simulink model "THREE_MPPTSTEST"  (R2016b)
settings: Solver=VariableStepAuto  StartTime=0.0  StopTime=0.5  RelTol=1e-3
values from neighbouring files (symbols this model uses):
  A = 1.3    [PV_module_Code.m]
  Isc = 8.61    [PV_module_Code.m]
  Ki = 0.002    [PV_module_Code.m]
  Kv = -0.32    [PV_module_Code.m]
  Ns = 60    [PV_module_Code.m]
  Rp = 415    [PV_module_Code.m]
  Rs = 0.22    [PV_module_Code.m]
  Voc = 37.41    [PV_module_Code.m]
undefined symbols (not defined in the file or in its folder): sigbuilder_block
libraries: powerlib x45, powerlib_meascontrol x3, fuzblock x1
settings Model: Creator=adria  LastModifiedBy=adria

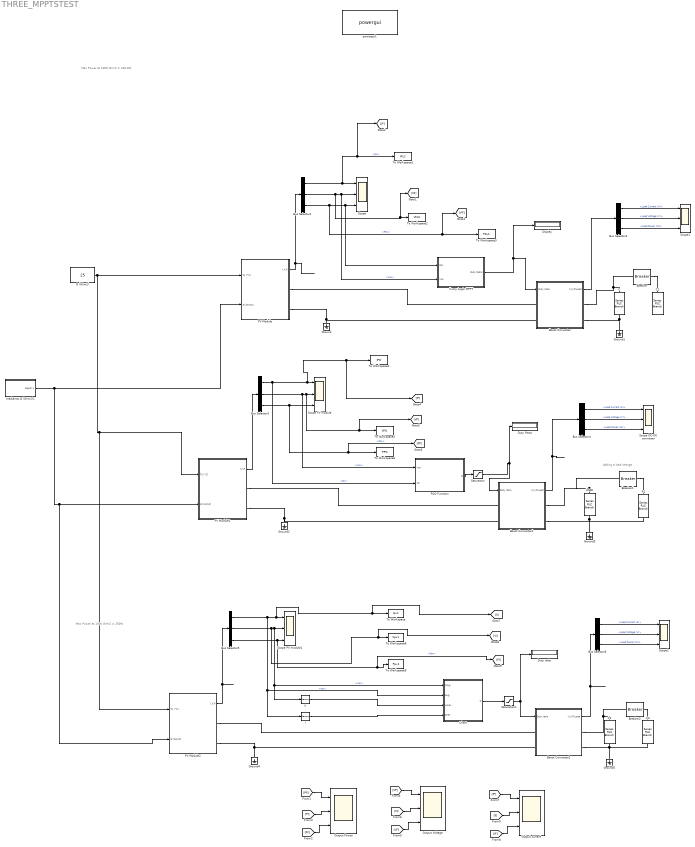
== system THREE_MPPTSTEST ==
  note: Max Power at 1000 W/m2 = 240.6W
  note: Adding a load change
  note: Max Power at 1000 W/m2 = 250W
  Boost Converter : Subsystem
  Boost Converter1 : Subsystem
  Boost Converter2 : Subsystem
  Breaker : powerlib/Elements/Breaker  InitialState=0  SwitchingTimes=[7]  External=off  BreakerResistance=0.00001  SnubberResistance=1e6  SnubberCapacitance=inf  Measurements=None  MoreParameters=on  NoBreakLoop=off
  Breaker1 : powerlib/Elements/Breaker  InitialState=0  SwitchingTimes=[5]  External=off  BreakerResistance=0.00001  SnubberResistance=1e6  SnubberCapacitance=inf  Measurements=None  MoreParameters=on  NoBreakLoop=off
  Breaker2 : powerlib/Elements/Breaker  InitialState=0  SwitchingTimes=[5]  External=off  BreakerResistance=0.00001  SnubberResistance=1e6  SnubberCapacitance=inf  Measurements=None  MoreParameters=on  NoBreakLoop=off
  Bus Selector1 : BusSelector  OutputSignals=Ipv,Vpv,Ppv
  Bus Selector2 : BusSelector  OutputSignals=Load Current (A),Load Voltage (V),Load Power (W)
  Bus Selector3 : BusSelector  OutputSignals=Ipv,Vpv,Ppv
  Bus Selector4 : BusSelector  OutputSignals=Load Current (A),Load Voltage (V),Load Power (W)
  Bus Selector5 : BusSelector  OutputSignals=Ipv,Vpv,Ppv
  Bus Selector6 : BusSelector  OutputSignals=Load Current (A),Load Voltage (V),Load Power (W)
  C : powerlib/Elements/Series RLC Branch  LConnTagsString=__new0  RConnTagsString=__new0  BranchType=R  Resistance=1000  Inductance=1e-3  SetiL0=off  InitialCurrent=0  Capacitance=19e-4  Setx0=off  InitialVoltage=0  Measurements=Branch voltage
  C1 : powerlib/Elements/Series RLC Branch  LConnTagsString=__new0  RConnTagsString=__new0  BranchType=R  Resistance=100  Inductance=1e-3  SetiL0=off  InitialCurrent=0  Capacitance=19e-4  Setx0=off  InitialVoltage=0  Measurements=Branch voltage
  C2 : powerlib/Elements/Series RLC Branch  LConnTagsString=__new0  RConnTagsString=__new0  BranchType=R  Resistance=100  Inductance=1e-3  SetiL0=off  InitialCurrent=0  Capacitance=19e-4  Setx0=off  InitialVoltage=0  Measurements=Branch voltage
  C3 : powerlib/Elements/Series RLC Branch  LConnTagsString=__new0  RConnTagsString=__new0  BranchType=R  Resistance=200  Inductance=1e-3  SetiL0=off  InitialCurrent=0  Capacitance=19e-4  Setx0=off  InitialVoltage=0  Measurements=Branch voltage
  Chart : Stateflow chart  TreatAsAtomicUnit=on
  Display : Display
  Duty Ratio : Display
  Duty ratio : Display
  Fuzzy Logic MPPT : Subsystem
  G (W/m2) : Constant  Value=25
  Ground{,1..5} (6 alike) : powerlib/Elements/Ground  LConnTagsString=a
  I : Memory
  Irradiance,G (W/m2)1 : Subsystem  Tag=STV Subsys  LoadFcn=sigbuilder_block('load');  StartFcn=sigbuilder_block('start');  StopFcn=sigbuilder_block('stop');  ClipboardFcn=sigbuilder_block('clipboard');  mask(Sigbuilder block){tuvar=[0:10]}
      mask help: Simulink:masks:SigbuilderBlock_MD
      mask init:
      | if ~strcmp(get_param(bdroot(gcbh),'SimulationStatus'),'stopped') tuvar = sigbuilder_block('maskInit'); end
      settings: CopyFcn=sigbuilder_block('copy');  DeleteFcn=sigbuilder_block('delete');  ModelCloseFcn=sigbuilder_block('modelClose');  PreSaveFcn=sigbuilder_block('preSave');  PauseFcn=sigbuilder_block('pause');  ContinueFcn=sigbuilder_block('continue');  NameChangeFcn=sigbuilder_block('namechange');  OpenFcn=sigbuilder_block('open',[484.8 30.6 470.4 453 ]);  CloseFcn=sigbuilder_block('close');
      mask Display: plot(0, 0, 100, 100,[2, 2, 32, 32, 2], [68, 8, 8, 68, 68],[32, 2], [38, 38], [32, 19, 2],[53, 60, 44], [32, 17, 17, 2],[16, 16, 31, 31]);txt = getActiveGroup(gcbh);text(2, 100, txt,'verticalAlignment', 'top');
  LOAD : powerlib/Elements/Series RLC Branch  LConnTagsString=__new0  RConnTagsString=__new0  BranchType=R  Resistance=100  Inductance=1e-3  SetiL0=off  InitialCurrent=0  Capacitance=19e-4  Setx0=off  InitialVoltage=0  Measurements=Branch voltage
  Output Power : Scope  NumInputPorts=3
  Output Voltage : Scope  NumInputPorts=3
  Output current : Scope  NumInputPorts=3
  P&O Function : MATLAB Function  TreatAsAtomicUnit=on
  PV Module : Subsystem
  PV Module1 : Subsystem
  PV Module2 : Subsystem
  R1 : powerlib/Elements/Series RLC Branch  LConnTagsString=__new0  RConnTagsString=__new0  BranchType=R  Resistance=200  Inductance=1e-3  SetiL0=off  InitialCurrent=0  Capacitance=19e-4  Setx0=off  InitialVoltage=0  Measurements=Branch voltage
  Saturation : Saturate  UpperLimit=1  LowerLimit=0.001  ZeroCross=off
  Saturation1 : Saturate  UpperLimit=1  LowerLimit=0.001  ZeroCross=off
  Scope : Scope  NumInputPorts=3
  Scope DC-DC converter : Scope  NumInputPorts=3
  Scope PV module1 : Scope  NumInputPorts=3
  Scope PV module : Scope  NumInputPorts=3
  Scope1 : Scope  NumInputPorts=3
  Scope2 : Scope  NumInputPorts=3
  To Workspace : ToWorkspace  VariableName=Ipv1  SampleTime=-1
  To Workspace1 : ToWorkspace  VariableName=IFLC  SampleTime=-1
  To Workspace2 : ToWorkspace  VariableName=VFLC  SampleTime=-1
  To Workspace3 : ToWorkspace  VariableName=PFLC  SampleTime=-1
  To Workspace4 : ToWorkspace  VariableName=IPO  SampleTime=-1
  To Workspace5 : ToWorkspace  VariableName=VPO  SampleTime=-1
  To Workspace6 : ToWorkspace  VariableName=PPO  SampleTime=-1
  To Workspace8 : ToWorkspace  VariableName=Vpv1  SampleTime=-1
  To Workspace9 : ToWorkspace  VariableName=Ppv1  SampleTime=-1
  V : Memory
  powergui1 : powerlib/powergui  Priority=1  SimulationMode=Discrete  SolverType=Tustin/Backward Euler (TBE)  SampleTime=0.000010  frequency=60  SPID=off  DisableSnubberDevices=off  DisableRonSwitches=off  DisableVfSwitches=off  SwTol=0  DisplayEquations=off  Interpol=off  ExternalGateDelay=off  methode=off  Ts=10  FunctionMessages=off  echomessages=off  HookPort=off  EnableUseOfTLC=off  x0status=blocks  frequencyindice=0  Pbase=100e6  ErrMax=1e-4  Iterations=50  UnitsV=kV  UnitsW=MW  buscounter=0  RestoreLinks=warning  ResistiveCurrentMeasurement=off  Frange=[0:2:500]  Ylog=off  Xlog=on  ShowGrid=off  save=off  variable=ZData  structure=0  ZoomFFT=off  StartTime=0.0  cycles=1  DisplayStyle=1  fundamental=60  FreqAxis=off  MaxFrequency=1000  frequencyindicesteady=1  RmsSteady=1  display=off
  wires:
  PV Module/1(I,V,P) -> Bus Selector1/1
  Bus Selector1/1 -> [IF], To Workspace1/1, Scope/1  "<Ipv>"
  Bus Selector1/2 -> [VF], To Workspace2/1, Fuzzy Logic MPPT/2(Vpv), Scope/2  "<Vpv>"
  Bus Selector1/3 -> [PF], To Workspace3/1, Fuzzy Logic MPPT/1(Ppv), Scope/3  "<Ppv>"
  Bus Selector2/1 -> Scope1/1  "<Load Current (A)>"
  Bus Selector2/2 -> Scope1/2  "<Load Voltage (V)>"
  Bus Selector2/3 -> Scope1/3  "<Load Power (W)>"
  Boost Converter/1((I,V,P)Load) -> Bus Selector2/1
  Fuzzy Logic MPPT/1(Duty Ratio) -> Display/1, Boost Converter/1("Duty ratio ")
  PV Module1/1(I,V,P) -> Bus Selector3/1
  Bus Selector3/1 -> P&O Function/2(Ipv), [IP], To Workspace4/1, Scope PV module/1  "<Ipv>"
  Bus Selector3/2 -> P&O Function/1(Vpv), [VP], To Workspace5/1, Scope PV module/2  "<Vpv>"
  Bus Selector3/3 -> [PP], To Workspace6/1, Scope PV module/3  "<Ppv>"
  Bus Selector4/1 -> Scope DC-DC converter/1  "<Load Current (A)>"
  Bus Selector4/2 -> Scope DC-DC converter/2  "<Load Voltage (V)>"
  Bus Selector4/3 -> Scope DC-DC converter/3  "<Load Power (W)>"
  Boost Converter1/1((I,V,P)Load) -> Bus Selector4/1
  P&O Function/1(D) -> Saturation/1
  Saturation/1 -> Duty Ratio/1, Boost Converter1/1("Duty ratio ")
  PV Module2/1(I,V,P) -> Bus Selector5/1
  Bus Selector5/1 -> I/1, Chart/2(Iavg), [II], To Workspace/1, Scope PV module1/1  "<Ipv>"
  Bus Selector6/1 -> Scope2/1  "<Load Current (A)>"
  Bus Selector6/2 -> Scope2/2  "<Load Voltage (V)>"
  Bus Selector6/3 -> Scope2/3  "<Load Power (W)>"
  Boost Converter2/1((I,V,P)Load) -> Bus Selector6/1
  Saturation1/1 -> Duty ratio/1, Boost Converter2/1("Duty ratio ")
  V/1 -> Chart/3(Vprev)
  I/1 -> Chart/4(Iprev)
  Chart/1(D) -> Saturation1/1
  Irradiance,G (W/m2)1/1(Signal 1) -> PV Module2/2(G (W/m2)), PV Module1/2(G (W/m2)), PV Module/2(G (W/m2))
  G (W/m2)/1 -> PV Module/1(Tc (°C)), PV Module2/1(Tc (°C)), PV Module1/1(Tc (°C))
  Bus Selector5/2 -> [VI], To Workspace8/1, V/1, Chart/1(Vavg), Scope PV module1/2  "<Vpv>"
  Bus Selector5/3 -> Scope PV module1/3, [PI], To Workspace9/1  "<Ppv>"
  [PF] -> Output Power/3
  [PI] -> Output Power/2
  [PP] -> Output Power/1
  [VF] -> Output Voltage/3
  [VI] -> Output Voltage/2
  [VP] -> Output Voltage/1
  [IF] -> Output current/3
  [II] -> Output current/2
  [IP] -> Output current/1
  connections:
  C/RConn1 -- Ground1/LConn1 -- Boost Converter/RConn2
  Boost Converter/LConn2 -- PV Module/RConn2 -- Ground/LConn1
  Breaker/LConn1 -- C/LConn1 -- Boost Converter/RConn1
  Breaker/RConn1 -- C1/LConn1
  PV Module/RConn1 -- Boost Converter/LConn1
  LOAD/RConn1 -- Boost Converter1/RConn2 -- Ground3/LConn1 -- R1/RConn1
  Ground2/LConn1 -- PV Module1/RConn2 -- Boost Converter1/LConn2
  LOAD/LConn1 -- Boost Converter1/RConn1 -- Breaker1/LConn1
  Breaker1/RConn1 -- R1/LConn1
  PV Module1/RConn1 -- Boost Converter1/LConn1
  Boost Converter2/RConn2 -- C2/RConn1 -- C3/RConn1 -- Ground5/LConn1
  PV Module2/RConn2 -- Boost Converter2/LConn2 -- Ground4/LConn1
  Breaker2/LConn1 -- C2/LConn1 -- Boost Converter2/RConn1
  Breaker2/RConn1 -- C3/LConn1
  PV Module2/RConn1 -- Boost Converter2/LConn1

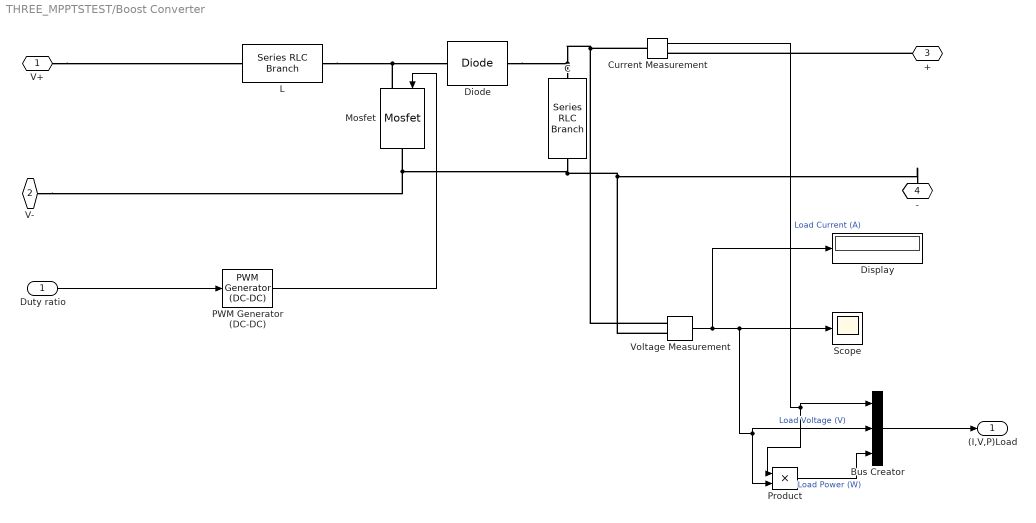
== system THREE_MPPTSTEST/Boost Converter ==
  "Duty ratio " : Inport
  Bus Creator : BusCreator  Inputs='Load Current (A)','Load Voltage (V)','Load Power (W)'
  C : powerlib/Elements/Series RLC Branch  LConnTagsString=__new0  RConnTagsString=__new0  BranchType=C  Resistance=1  Inductance=1e-3  SetiL0=off  InitialCurrent=0  Capacitance=50e-5  Setx0=off  InitialVoltage=0  Measurements=None
  Current Measurement : powerlib/Measurements/Current Measurement  PhasorSimulation=off  OutputType=Complex  PSBequivalent=0
  Diode : powerlib/Power Electronics/Diode  Ron=0.0001  Lon=0  Vf=0.8  IC=0  UseSnubber=off  Rs=500  Cs=250e-9  Measurements=off
  Display : Display
  L : powerlib/Elements/Series RLC Branch  LConnTagsString=__new0  RConnTagsString=__new0  BranchType=L  Resistance=1  Inductance=1e-3  SetiL0=off  InitialCurrent=0  Capacitance=1e-6  Setx0=off  InitialVoltage=0  Measurements=None
  Mosfet : powerlib/Power Electronics/Mosfet  Ron=0.0001  Lon=0  Rd=0.0001  Vfd=0  IC=0  Rs=1e5  Cs=inf  Measurements=off
  PWM Generator (DC-DC) : powerlib_meascontrol/Pulse & Signal Generators/PWM Generator (DC-DC)  Fsw=1000  Ts=0
  Product : Product
  Scope : Scope
  Voltage Measurement : powerlib/Measurements/Voltage Measurement  PhasorSimulation=off  OutputType=Complex  PSBequivalent=0
  V+ : PMIOPort  Port=1  Side=Left
  V- : PMIOPort  Port=2  Side=Left
  + : PMIOPort  Port=3  Side=Right
  - : PMIOPort  Port=4  Side=Right
  (I,V,P)Load : Outport
  wires:
  PWM Generator (DC-DC)/1 -> Mosfet/1
  Voltage Measurement/1 -> Display/1, Product/2, Bus Creator/2, Scope/1  "Load Voltage (V)"
  "Duty ratio "/1 -> PWM Generator (DC-DC)/1
  Current Measurement/1 -> Product/1, Bus Creator/1  "Load Current (A)"
  Product/1 -> Bus Creator/3  "Load Power (W)"
  Bus Creator/1 -> (I,V,P)Load/1
  connections:
  V+/RConn1 -- L/LConn1
  L/RConn1 -- Mosfet/LConn1 -- Diode/LConn1
  +/RConn1 -- Current Measurement/RConn1
  -/RConn1 -- Voltage Measurement/LConn2 -- V-/RConn1 -- Mosfet/RConn1 -- C/RConn1
  Diode/RConn1 -- Current Measurement/LConn1 -- Voltage Measurement/LConn1 -- C/LConn1

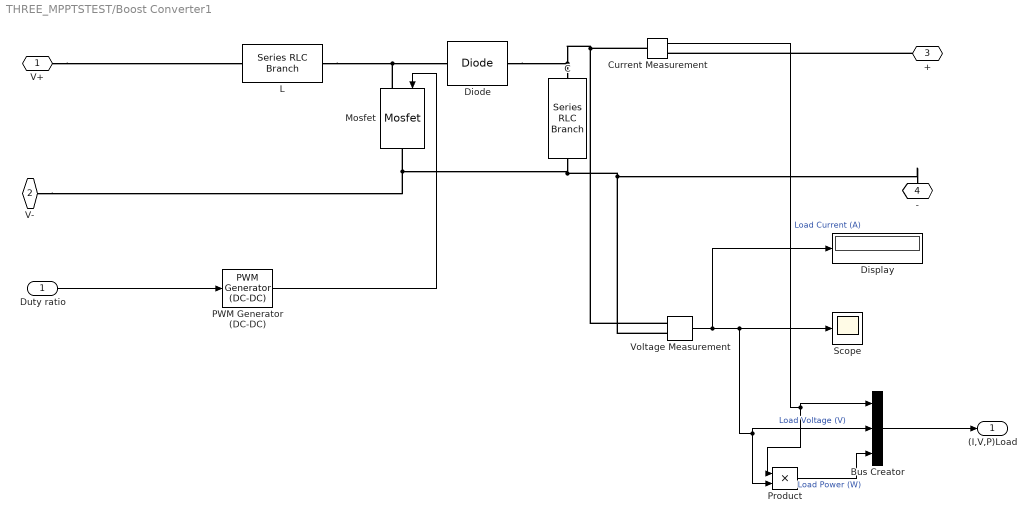
== system THREE_MPPTSTEST/Boost Converter1 ==
  "Duty ratio " : Inport
  Bus Creator : BusCreator  Inputs='Load Current (A)','Load Voltage (V)','Load Power (W)'
  C : powerlib/Elements/Series RLC Branch  LConnTagsString=__new0  RConnTagsString=__new0  BranchType=C  Resistance=1  Inductance=1e-3  SetiL0=off  InitialCurrent=0  Capacitance=50e-5  Setx0=off  InitialVoltage=0  Measurements=None
  Current Measurement : powerlib/Measurements/Current Measurement  PhasorSimulation=off  OutputType=Complex  PSBequivalent=0
  Diode : powerlib/Power Electronics/Diode  Ron=0.0001  Lon=0  Vf=0.8  IC=0  UseSnubber=off  Rs=500  Cs=250e-9  Measurements=off
  Display : Display
  L : powerlib/Elements/Series RLC Branch  LConnTagsString=__new0  RConnTagsString=__new0  BranchType=L  Resistance=1  Inductance=1e-3  SetiL0=off  InitialCurrent=0  Capacitance=1e-6  Setx0=off  InitialVoltage=0  Measurements=None
  Mosfet : powerlib/Power Electronics/Mosfet  Ron=0.0001  Lon=0  Rd=0.0001  Vfd=0  IC=0  Rs=1e5  Cs=inf  Measurements=off
  PWM Generator (DC-DC) : powerlib_meascontrol/Pulse & Signal Generators/PWM Generator (DC-DC)  Fsw=1000  Ts=0
  Product : Product
  Scope : Scope
  Voltage Measurement : powerlib/Measurements/Voltage Measurement  PhasorSimulation=off  OutputType=Complex  PSBequivalent=0
  V+ : PMIOPort  Port=1  Side=Left
  V- : PMIOPort  Port=2  Side=Left
  + : PMIOPort  Port=3  Side=Right
  - : PMIOPort  Port=4  Side=Right
  (I,V,P)Load : Outport
  wires:
  PWM Generator (DC-DC)/1 -> Mosfet/1
  Voltage Measurement/1 -> Display/1, Product/2, Bus Creator/2, Scope/1  "Load Voltage (V)"
  "Duty ratio "/1 -> PWM Generator (DC-DC)/1
  Current Measurement/1 -> Product/1, Bus Creator/1  "Load Current (A)"
  Product/1 -> Bus Creator/3  "Load Power (W)"
  Bus Creator/1 -> (I,V,P)Load/1
  connections:
  V+/RConn1 -- L/LConn1
  L/RConn1 -- Mosfet/LConn1 -- Diode/LConn1
  +/RConn1 -- Current Measurement/RConn1
  -/RConn1 -- Voltage Measurement/LConn2 -- V-/RConn1 -- Mosfet/RConn1 -- C/RConn1
  Diode/RConn1 -- Current Measurement/LConn1 -- Voltage Measurement/LConn1 -- C/LConn1

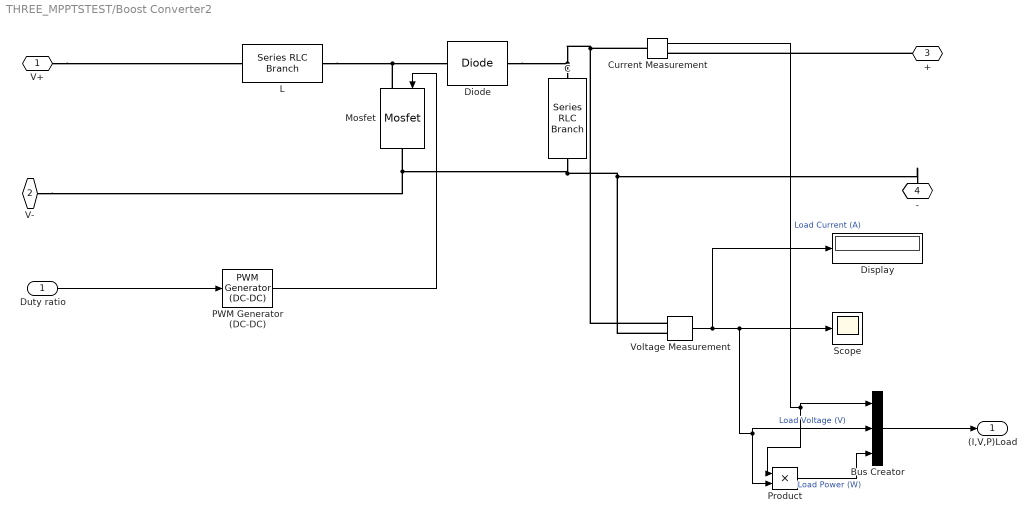
== system THREE_MPPTSTEST/Boost Converter2 ==
  "Duty ratio " : Inport
  Bus Creator : BusCreator  Inputs='Load Current (A)','Load Voltage (V)','Load Power (W)'
  C : powerlib/Elements/Series RLC Branch  LConnTagsString=__new0  RConnTagsString=__new0  BranchType=C  Resistance=1  Inductance=1e-3  SetiL0=off  InitialCurrent=0  Capacitance=50e-5  Setx0=off  InitialVoltage=0  Measurements=None
  Current Measurement : powerlib/Measurements/Current Measurement  PhasorSimulation=off  OutputType=Complex  PSBequivalent=0
  Diode : powerlib/Power Electronics/Diode  Ron=0.001  Lon=0  Vf=0.8  IC=0  UseSnubber=off  Rs=500  Cs=250e-9  Measurements=off
  Display : Display
  L : powerlib/Elements/Series RLC Branch  LConnTagsString=__new0  RConnTagsString=__new0  BranchType=L  Resistance=1  Inductance=1e-3  SetiL0=off  InitialCurrent=0  Capacitance=1e-6  Setx0=off  InitialVoltage=0  Measurements=None
  Mosfet : powerlib/Power Electronics/Mosfet  Ron=0.0001  Lon=0  Rd=0.0001  Vfd=0  IC=0  Rs=1e5  Cs=inf  Measurements=off
  PWM Generator (DC-DC) : powerlib_meascontrol/Pulse & Signal Generators/PWM Generator (DC-DC)  Fsw=1000  Ts=0
  Product : Product
  Scope : Scope
  Voltage Measurement : powerlib/Measurements/Voltage Measurement  PhasorSimulation=off  OutputType=Complex  PSBequivalent=0
  V+ : PMIOPort  Port=1  Side=Left
  V- : PMIOPort  Port=2  Side=Left
  + : PMIOPort  Port=3  Side=Right
  - : PMIOPort  Port=4  Side=Right
  (I,V,P)Load : Outport
  wires:
  PWM Generator (DC-DC)/1 -> Mosfet/1
  Voltage Measurement/1 -> Display/1, Product/2, Bus Creator/2, Scope/1  "Load Voltage (V)"
  "Duty ratio "/1 -> PWM Generator (DC-DC)/1
  Current Measurement/1 -> Product/1, Bus Creator/1  "Load Current (A)"
  Product/1 -> Bus Creator/3  "Load Power (W)"
  Bus Creator/1 -> (I,V,P)Load/1
  connections:
  V+/RConn1 -- L/LConn1
  L/RConn1 -- Mosfet/LConn1 -- Diode/LConn1
  +/RConn1 -- Current Measurement/RConn1
  -/RConn1 -- Voltage Measurement/LConn2 -- V-/RConn1 -- Mosfet/RConn1 -- C/RConn1
  Diode/RConn1 -- Current Measurement/LConn1 -- Voltage Measurement/LConn1 -- C/LConn1

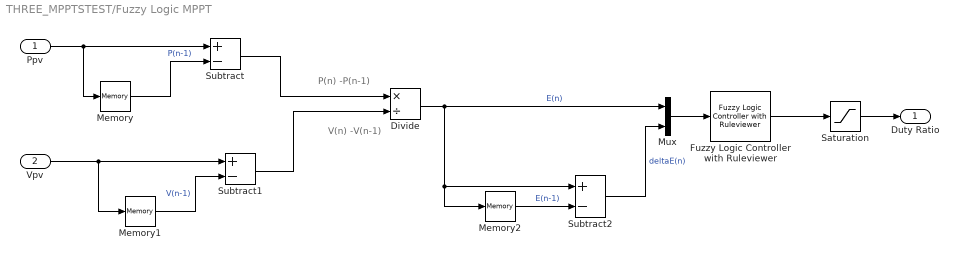
== system THREE_MPPTSTEST/Fuzzy Logic MPPT ==
  note: P(n) -P(n-1)
  note: V(n) -V(n-1)
  Ppv : Inport
  Vpv : Inport  Port=2
  Divide : Product  Inputs=*/
  Fuzzy Logic Controller with Ruleviewer : fuzblock/Fuzzy Logic  Controller  with Ruleviewer  fismatrix=MPPT8  Ts=1
  Memory : Memory  InheritSampleTime=on
  Memory1 : Memory  InheritSampleTime=on
  Memory2 : Memory
  Mux : Mux  Inputs=2
  Saturation : Saturate  UpperLimit=1  LowerLimit=0  LinearizeAsGain=off  ZeroCross=off
  Subtract : Sum  Inputs=+-
  Subtract1 : Sum  Inputs=+-
  Subtract2 : Sum  Inputs=+-
  Duty Ratio : Outport
  wires:
  Ppv/1 -> Subtract/1, Memory/1
  Mux/1 -> Fuzzy Logic Controller with Ruleviewer/1
  Divide/1 -> Subtract2/1, Memory2/1, Mux/1  "E(n)"
  Memory2/1 -> Subtract2/2  "E(n-1)"
  Subtract2/1 -> Mux/2  "deltaE(n)"
  Memory/1 -> Subtract/2  "P(n-1)"
  Vpv/1 -> Memory1/1, Subtract1/1
  Memory1/1 -> Subtract1/2  "V(n-1)"
  Saturation/1 -> Duty Ratio/1
  Subtract1/1 -> Divide/2
  Subtract/1 -> Divide/1
  Fuzzy Logic Controller with Ruleviewer/1 -> Saturation/1

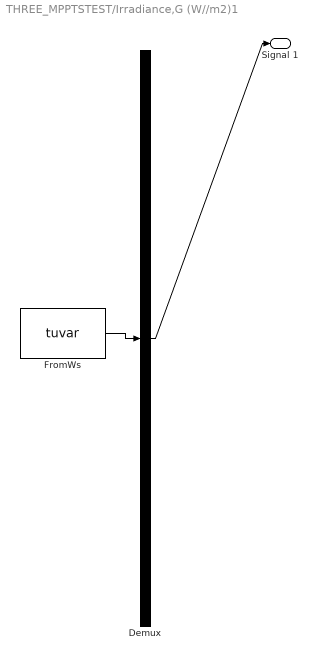
== system THREE_MPPTSTEST/Irradiance,G (W//m2)1 ==
  Demux : Demux  Tag=STV Demux  Outputs=1
  FromWs : FromWorkspace  Tag=STV FromWs  VariableName=tuvar  SampleTime=0
      SigBuilderData=|
      | common.afterFinalStr = 'Extrapolate'
      | common.sampleTime = 0
      | dataSet.timeRange = [0 10]
      | dataSet.name = 'Irradiance Variation Pattern'
      | sbobj.Groups.Name = 'Irradiance Variation Pattern'
      | sbobj.Groups.Signals.Name = 'Signal 1'
      | sbobj.Groups.Signals.XData = [0 0.2 0.2 0.3 0.3 0.8 0.8 0.9 2.4 2.4 3.6 3.6 10]
      | sbobj.Groups.Signals.YData = [1000 1000 300 300 1000 1000 995 995 995 575 1 0 0]
  Signal 1 : Outport  Tag=STV Outport
  wires:
  FromWs/1 -> Demux/1
  Demux/1 -> Signal 1/1

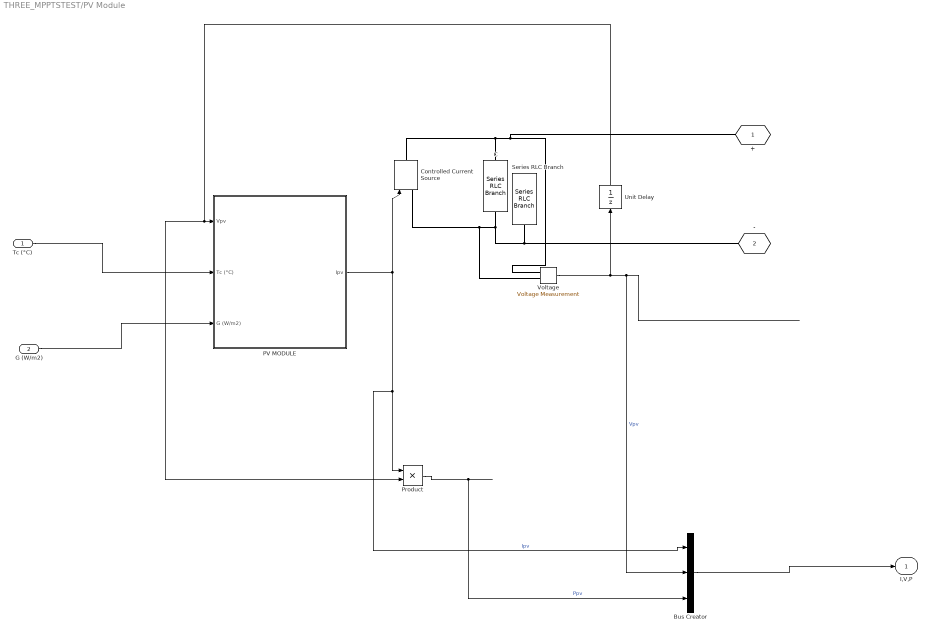
== system THREE_MPPTSTEST/PV Module ==
  Tc (°C) : Inport
  G (W/m2) : Inport  Port=2
  Bus Creator : BusCreator  Inputs='Ipv','Vpv','Ppv'
  C : powerlib/Elements/Series RLC Branch  LConnTagsString=__new0  RConnTagsString=__new0  BranchType=C  Resistance=10  Inductance=1e-3  SetiL0=off  InitialCurrent=0  Capacitance=30e-4  Setx0=off  InitialVoltage=0  Measurements=Branch voltage
  Controlled Current Source : powerlib/Electrical Sources/Controlled Current Source  Initialize=on  Source_Type=DC  Amplitude=0  Phase=0  Frequency=0  Measurements=None
  PV MODULE : Subsystem
  Product : Product
  Series RLC Branch : powerlib/Elements/Series RLC Branch  LConnTagsString=__new0  RConnTagsString=__new0  BranchType=R  Resistance=1000  Inductance=1e-3  SetiL0=off  InitialCurrent=0  Capacitance=1e-6  Setx0=off  InitialVoltage=0  Measurements=None
  Unit Delay : UnitDelay  SampleTime=-1
  "Voltage " : powerlib/Measurements/Voltage Measurement  PhasorSimulation=off  OutputType=Complex  PSBequivalent=0
  + : PMIOPort  Port=1  Side=Right
  - : PMIOPort  Port=2  Side=Right
  I,V,P : Outport
  wires:
  Product/1 -> Bus Creator/3  "Ppv"
  Tc (°C)/1 -> PV MODULE/2("Tc (°C) ")
  G (W/m2)/1 -> PV MODULE/3(G (W/m2))
  "Voltage "/1 -> Unit Delay/1, Bus Creator/2  "Vpv"
  PV MODULE/1(Ipv) -> Controlled Current Source/1, Bus Creator/1, Product/1  "Ipv"
  Bus Creator/1 -> I,V,P/1
  Unit Delay/1 -> Product/2, PV MODULE/1(Vpv)
  connections:
  Controlled Current Source/LConn1 -- Series RLC Branch/RConn1 -- -/RConn1 -- C/RConn1 -- "Voltage "/LConn2
  Controlled Current Source/RConn1 -- C/LConn1 -- "Voltage "/LConn1 -- +/RConn1

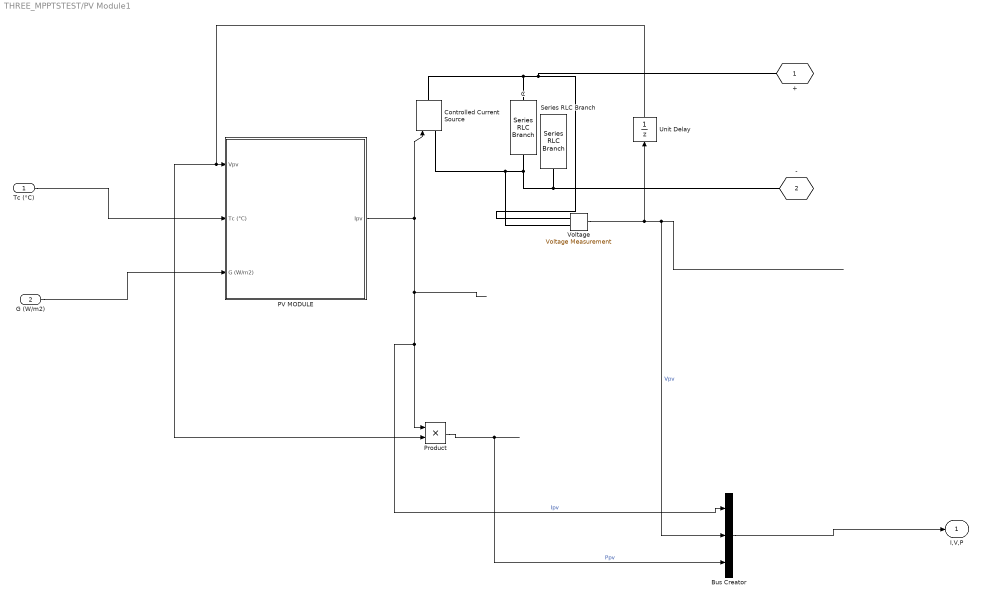
== system THREE_MPPTSTEST/PV Module1 ==
  Tc (°C) : Inport
  G (W/m2) : Inport  Port=2
  Bus Creator : BusCreator  Inputs='Ipv','Vpv','Ppv'
  C : powerlib/Elements/Series RLC Branch  LConnTagsString=__new0  RConnTagsString=__new0  BranchType=C  Resistance=10  Inductance=1e-3  SetiL0=off  InitialCurrent=0  Capacitance=30e-4  Setx0=off  InitialVoltage=0  Measurements=Branch voltage
  Controlled Current Source : powerlib/Electrical Sources/Controlled Current Source  Initialize=on  Source_Type=AC  Amplitude=0  Phase=0  Frequency=0  Measurements=None
  PV MODULE : Subsystem
  Product : Product
  Series RLC Branch : powerlib/Elements/Series RLC Branch  LConnTagsString=__new0  RConnTagsString=__new0  BranchType=R  Resistance=1000  Inductance=1e-3  SetiL0=off  InitialCurrent=0  Capacitance=1e-6  Setx0=off  InitialVoltage=0  Measurements=None
  Unit Delay : UnitDelay  SampleTime=-1
  "Voltage " : powerlib/Measurements/Voltage Measurement  PhasorSimulation=off  OutputType=Complex  PSBequivalent=0
  + : PMIOPort  Port=1  Side=Right
  - : PMIOPort  Port=2  Side=Right
  I,V,P : Outport
  wires:
  Product/1 -> Bus Creator/3  "Ppv"
  Tc (°C)/1 -> PV MODULE/2("Tc (°C) ")
  G (W/m2)/1 -> PV MODULE/3(G (W/m2))
  "Voltage "/1 -> Unit Delay/1, Bus Creator/2  "Vpv"
  PV MODULE/1(Ipv) -> Controlled Current Source/1, Bus Creator/1, Product/1  "Ipv"
  Bus Creator/1 -> I,V,P/1
  Unit Delay/1 -> Product/2, PV MODULE/1(Vpv)
  connections:
  Controlled Current Source/LConn1 -- Series RLC Branch/RConn1 -- -/RConn1 -- C/RConn1 -- "Voltage "/LConn2
  Controlled Current Source/RConn1 -- C/LConn1 -- "Voltage "/LConn1 -- +/RConn1

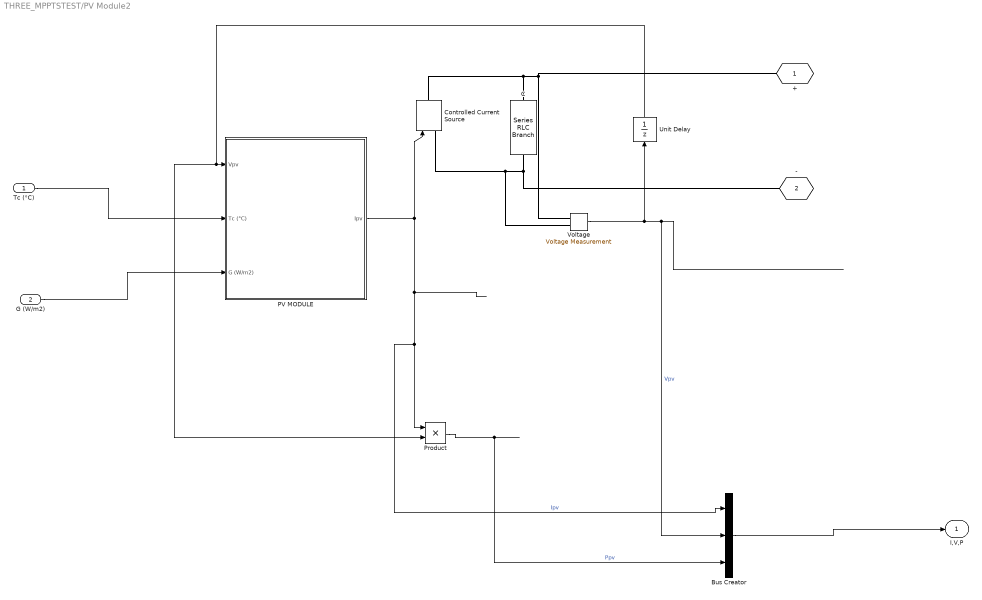
== system THREE_MPPTSTEST/PV Module2 ==
  Tc (°C) : Inport
  G (W/m2) : Inport  Port=2
  Bus Creator : BusCreator  Inputs='Ipv','Vpv','Ppv'
  C : powerlib/Elements/Series RLC Branch  LConnTagsString=__new0  RConnTagsString=__new0  BranchType=C  Resistance=10  Inductance=1e-3  SetiL0=off  InitialCurrent=0  Capacitance=30e-4  Setx0=off  InitialVoltage=0  Measurements=Branch voltage
  Controlled Current Source : powerlib/Electrical Sources/Controlled Current Source  Initialize=on  Source_Type=AC  Amplitude=0  Phase=0  Frequency=0  Measurements=None
  PV MODULE : Subsystem
  Product : Product
  Unit Delay : UnitDelay  SampleTime=-1
  "Voltage " : powerlib/Measurements/Voltage Measurement  PhasorSimulation=off  OutputType=Complex  PSBequivalent=0
  + : PMIOPort  Port=1  Side=Right
  - : PMIOPort  Port=2  Side=Right
  I,V,P : Outport
  wires:
  Product/1 -> Bus Creator/3  "Ppv"
  Tc (°C)/1 -> PV MODULE/2("Tc (°C) ")
  G (W/m2)/1 -> PV MODULE/3(G (W/m2))
  "Voltage "/1 -> Unit Delay/1, Bus Creator/2  "Vpv"
  PV MODULE/1(Ipv) -> Controlled Current Source/1, Bus Creator/1, Product/1  "Ipv"
  Bus Creator/1 -> I,V,P/1
  Unit Delay/1 -> Product/2, PV MODULE/1(Vpv)
  connections:
  Controlled Current Source/LConn1 -- -/RConn1 -- C/RConn1 -- "Voltage "/LConn2
  Controlled Current Source/RConn1 -- C/LConn1 -- +/RConn1 -- "Voltage "/LConn1

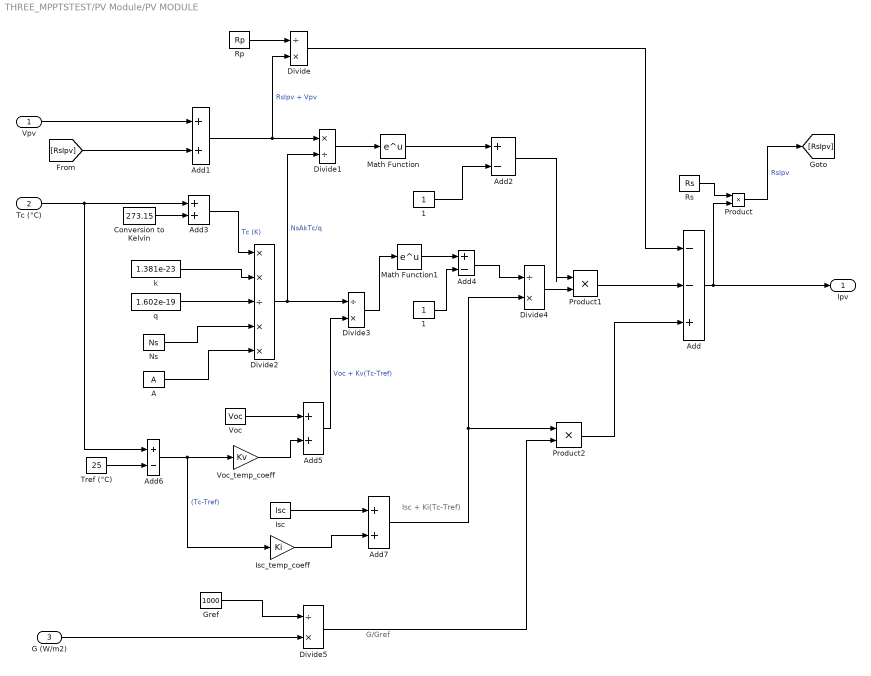
== system THREE_MPPTSTEST/PV Module/PV MODULE ==
  note: G/Gref
  note: Isc + Ki(Tc-Tref)
  Vpv : Inport
  "Tc (°C) " : Inport  Port=2
  G (W/m2) : Inport  Port=3
  " 1" : Constant
  " Gref " : Constant  Value=1000
  " Tref (°C)" : Constant  Value=25
  " Voc" : Constant  Value=Voc
  1 : Constant
  A : Constant  Value=A
  Add : Sum  Inputs=--+
  Add{1,3,5,7} (4 alike) : Sum
  Add2 : Sum  Inputs=+-
  Add4 : Sum  Inputs=+-
  Add6 : Sum  Inputs=+-
  Conversion to Kelvin : Constant  Value=273.15
  Divide{,3..5} (4 alike) : Product  Inputs=/*
  Divide1 : Product  Inputs=*/
  Divide2 : Product  Inputs=**/**
  Isc : Constant  Value=Isc
  "Isc_temp_coeff " : Gain  Gain=Ki
  Math Function : Math  SaturateOnIntegerOverflow=on
  Math Function1 : Math  SaturateOnIntegerOverflow=on
  Ns : Constant  Value=Ns
  Product : Product
  Product1 : Product
  Product2 : Product
  Rp : Constant  Value=Rp
  Rs : Constant  Value=Rs
  Voc_temp_coeff : Gain  Gain=Kv
  k : Constant  Value=1.381e-23
  "q " : Constant  Value=1.602e-19
  Ipv : Outport
  wires:
  A/1 -> Divide2/5
  Vpv/1 -> Add1/1
  Rp/1 -> Divide/1
  Add/1 -> Ipv/1, Product/2
  Product/1 -> [RsIpv]  "RsIpv"
  Divide/1 -> Add/1
  Add1/1 -> Divide1/1, Divide/2  "RsIpv + Vpv"
  Rs/1 -> Product/1
  Product2/1 -> Add/3
  Divide2/1 -> Divide3/1, Divide1/2  "NsAkTc/q"
  k/1 -> Divide2/2
  Math Function1/1 -> Add4/1
  " Voc"/1 -> Add5/1
  Divide4/1 -> Product1/2
  Add2/1 -> Product1/1
  Math Function/1 -> Add2/1
  Divide3/1 -> Math Function1/1
  "q "/1 -> Divide2/3
  Add6/1 -> "Isc_temp_coeff "/1, Voc_temp_coeff/1  "(Tc-Tref)"
  " 1"/1 -> Add4/2
  Isc/1 -> Add7/1
  Add7/1 -> Product2/1, Divide4/2
  "Tc (°C) "/1 -> Add6/1, Add3/1
  Add4/1 -> Divide4/1
  Product1/1 -> Add/2
  Divide5/1 -> Product2/2
  Conversion to Kelvin/1 -> Add3/2
  Add5/1 -> Divide3/2  "Voc + Kv(Tc-Tref)"
  "Isc_temp_coeff "/1 -> Add7/2
  Divide1/1 -> Math Function/1
  " Gref "/1 -> Divide5/1
  " Tref (°C)"/1 -> Add6/2
  G (W/m2)/1 -> Divide5/2
  Voc_temp_coeff/1 -> Add5/2
  Add3/1 -> Divide2/1  "Tc (K)"
  Ns/1 -> Divide2/4
  1/1 -> Add2/2
  [RsIpv] -> Add1/2

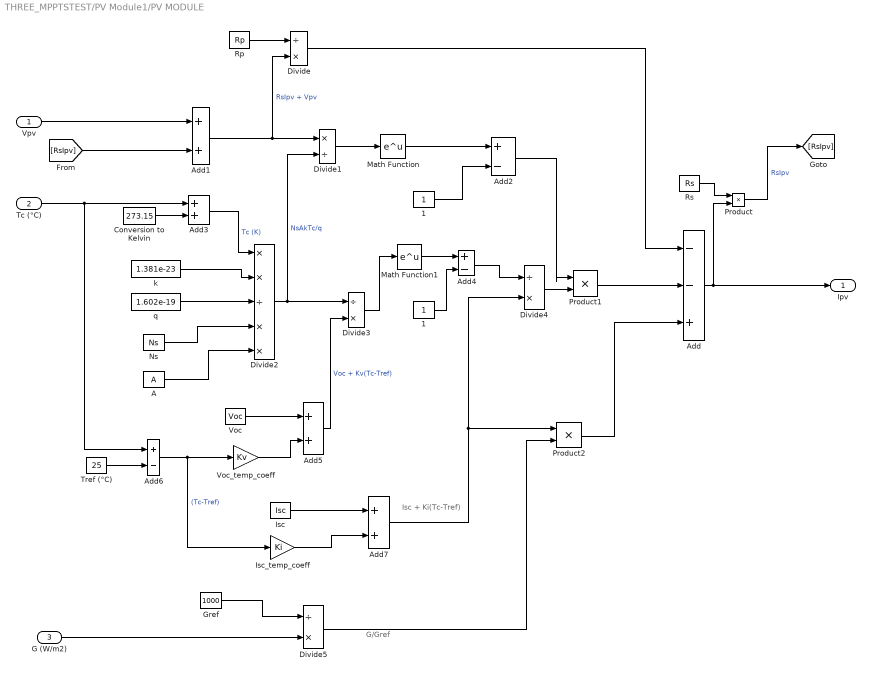
== system THREE_MPPTSTEST/PV Module1/PV MODULE ==
  note: G/Gref
  note: Isc + Ki(Tc-Tref)
  Vpv : Inport
  "Tc (°C) " : Inport  Port=2
  G (W/m2) : Inport  Port=3
  " 1" : Constant
  " Gref " : Constant  Value=1000
  " Tref (°C)" : Constant  Value=25
  " Voc" : Constant  Value=Voc
  1 : Constant
  A : Constant  Value=A
  Add : Sum  Inputs=--+
  Add{1,3,5,7} (4 alike) : Sum
  Add2 : Sum  Inputs=+-
  Add4 : Sum  Inputs=+-
  Add6 : Sum  Inputs=+-
  Conversion to Kelvin : Constant  Value=273.15
  Divide{,3..5} (4 alike) : Product  Inputs=/*
  Divide1 : Product  Inputs=*/
  Divide2 : Product  Inputs=**/**
  Isc : Constant  Value=Isc
  "Isc_temp_coeff " : Gain  Gain=Ki
  Math Function : Math  SaturateOnIntegerOverflow=on
  Math Function1 : Math  SaturateOnIntegerOverflow=on
  Ns : Constant  Value=Ns
  Product : Product
  Product1 : Product
  Product2 : Product
  Rp : Constant  Value=Rp
  Rs : Constant  Value=Rs
  Voc_temp_coeff : Gain  Gain=Kv
  k : Constant  Value=1.381e-23
  "q " : Constant  Value=1.602e-19
  Ipv : Outport
  wires:
  A/1 -> Divide2/5
  Vpv/1 -> Add1/1
  Rp/1 -> Divide/1
  Add/1 -> Ipv/1, Product/2
  Product/1 -> [RsIpv]  "RsIpv"
  Divide/1 -> Add/1
  Add1/1 -> Divide1/1, Divide/2  "RsIpv + Vpv"
  Rs/1 -> Product/1
  Product2/1 -> Add/3
  Divide2/1 -> Divide3/1, Divide1/2  "NsAkTc/q"
  k/1 -> Divide2/2
  Math Function1/1 -> Add4/1
  " Voc"/1 -> Add5/1
  Divide4/1 -> Product1/2
  Add2/1 -> Product1/1
  Math Function/1 -> Add2/1
  Divide3/1 -> Math Function1/1
  "q "/1 -> Divide2/3
  Add6/1 -> "Isc_temp_coeff "/1, Voc_temp_coeff/1  "(Tc-Tref)"
  " 1"/1 -> Add4/2
  Isc/1 -> Add7/1
  Add7/1 -> Product2/1, Divide4/2
  "Tc (°C) "/1 -> Add6/1, Add3/1
  Add4/1 -> Divide4/1
  Product1/1 -> Add/2
  Divide5/1 -> Product2/2
  Conversion to Kelvin/1 -> Add3/2
  Add5/1 -> Divide3/2  "Voc + Kv(Tc-Tref)"
  "Isc_temp_coeff "/1 -> Add7/2
  Divide1/1 -> Math Function/1
  " Gref "/1 -> Divide5/1
  " Tref (°C)"/1 -> Add6/2
  G (W/m2)/1 -> Divide5/2
  Voc_temp_coeff/1 -> Add5/2
  Add3/1 -> Divide2/1  "Tc (K)"
  Ns/1 -> Divide2/4
  1/1 -> Add2/2
  [RsIpv] -> Add1/2

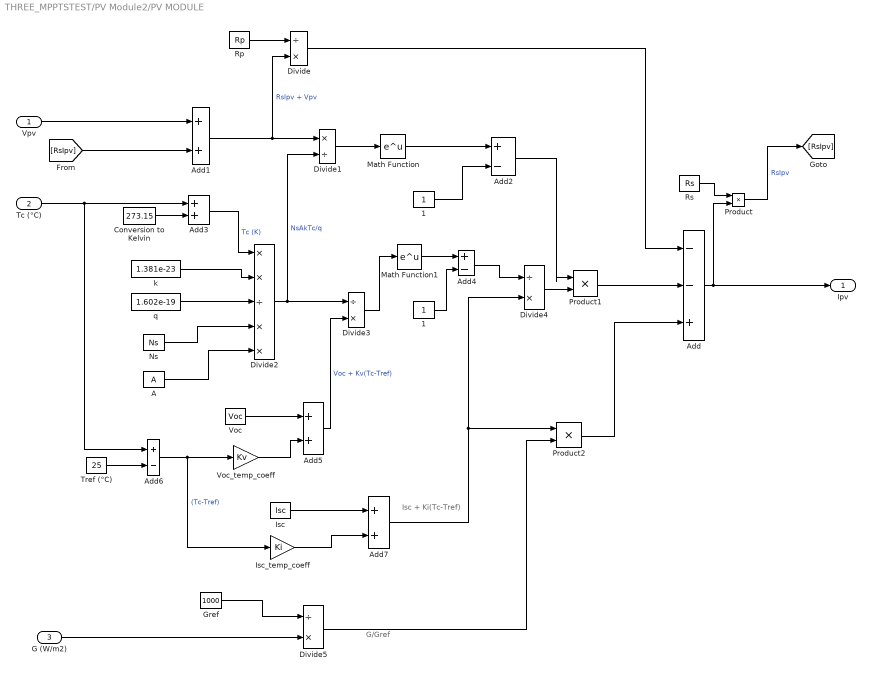
== system THREE_MPPTSTEST/PV Module2/PV MODULE ==
  note: G/Gref
  note: Isc + Ki(Tc-Tref)
  Vpv : Inport
  "Tc (°C) " : Inport  Port=2
  G (W/m2) : Inport  Port=3
  " 1" : Constant
  " Gref " : Constant  Value=1000
  " Tref (°C)" : Constant  Value=25
  " Voc" : Constant  Value=Voc
  1 : Constant
  A : Constant  Value=A
  Add : Sum  Inputs=--+
  Add{1,3,5,7} (4 alike) : Sum
  Add2 : Sum  Inputs=+-
  Add4 : Sum  Inputs=+-
  Add6 : Sum  Inputs=+-
  Conversion to Kelvin : Constant  Value=273.15
  Divide{,3..5} (4 alike) : Product  Inputs=/*
  Divide1 : Product  Inputs=*/
  Divide2 : Product  Inputs=**/**
  Isc : Constant  Value=Isc
  "Isc_temp_coeff " : Gain  Gain=Ki
  Math Function : Math  SaturateOnIntegerOverflow=on
  Math Function1 : Math  SaturateOnIntegerOverflow=on
  Ns : Constant  Value=Ns
  Product : Product
  Product1 : Product
  Product2 : Product
  Rp : Constant  Value=Rp
  Rs : Constant  Value=Rs
  Voc_temp_coeff : Gain  Gain=Kv
  k : Constant  Value=1.381e-23
  "q " : Constant  Value=1.602e-19
  Ipv : Outport
  wires:
  A/1 -> Divide2/5
  Vpv/1 -> Add1/1
  Rp/1 -> Divide/1
  Add/1 -> Ipv/1, Product/2
  Product/1 -> [RsIpv]  "RsIpv"
  Divide/1 -> Add/1
  Add1/1 -> Divide1/1, Divide/2  "RsIpv + Vpv"
  Rs/1 -> Product/1
  Product2/1 -> Add/3
  Divide2/1 -> Divide3/1, Divide1/2  "NsAkTc/q"
  k/1 -> Divide2/2
  Math Function1/1 -> Add4/1
  " Voc"/1 -> Add5/1
  Divide4/1 -> Product1/2
  Add2/1 -> Product1/1
  Math Function/1 -> Add2/1
  Divide3/1 -> Math Function1/1
  "q "/1 -> Divide2/3
  Add6/1 -> "Isc_temp_coeff "/1, Voc_temp_coeff/1  "(Tc-Tref)"
  " 1"/1 -> Add4/2
  Isc/1 -> Add7/1
  Add7/1 -> Product2/1, Divide4/2
  "Tc (°C) "/1 -> Add6/1, Add3/1
  Add4/1 -> Divide4/1
  Product1/1 -> Add/2
  Divide5/1 -> Product2/2
  Conversion to Kelvin/1 -> Add3/2
  Add5/1 -> Divide3/2  "Voc + Kv(Tc-Tref)"
  "Isc_temp_coeff "/1 -> Add7/2
  Divide1/1 -> Math Function/1
  " Gref "/1 -> Divide5/1
  " Tref (°C)"/1 -> Add6/2
  G (W/m2)/1 -> Divide5/2
  Voc_temp_coeff/1 -> Add5/2
  Add3/1 -> Divide2/1  "Tc (K)"
  Ns/1 -> Divide2/4
  1/1 -> Add2/2
  [RsIpv] -> Add1/2

== matlab function THREE_MPPTSTEST/P&O Function ==
  data: Vpv input; D output; Ipv input
function D = PO_Algorithm(Vpv,Ipv)
%P&O algoritm implmentation designed to operate 
%with Boost converter
%************************************
%Created by Joseph Adriano Nemours

%Define Inernal Values for the power nad voltage 
%a persistent variables
persistent Dprev Pprev Vprev

%Initialise the internal vlaues for the voltage 
%and power on the first pass (ot iteration)
if isempty (Dprev)
    Dprev = 0.8;
    Vprev = 30;
    Pprev = 250;
end

%Initialise algoritm parameters
deltaD = 0.001;

%Calculate measured array power
Ppv = Ipv * Vpv;

%Increase or decrease duty cycle 
%based on conditions
if (Ppv-Pprev)~= 0
    if (Ppv-Pprev) > 0
        if (Vpv-Vprev) > 0
            D = Dprev - deltaD;
        else 
            D = Dprev + deltaD;
        end
    else
        if (Vpv-Vprev) > 0
                D = Dprev + deltaD;
        else
            D = Dprev - deltaD;
        end
    end
else
    D = Dprev;
end
if D >= 0.8 || D<= 0
 D=Dprev;
end

%Update internal value of Duty ratio
Dprev = D;
Pprev = Ppv;
Vprev = Vpv;

== stateflow chart THREE_MPPTSTEST/Chart ==
  state DEFINE
    entry: D=0.8;
  state SAMPLEandCALCULATE
    entry:
    deltaV = Vavg-Vprev;
    deltaI = Iavg - Iprev;
    d=D;
  state INCREMENT_D
    entry:
    d = d + 0.001;
  state DECREMENT_D
    entry:
    d = d - 0.001;
  state RETURN
    entry:
    D = d;
  (default) -> DEFINE
  RETURN -> SAMPLEandCALCULATE
  DEFINE -> SAMPLEandCALCULATE
  SAMPLEandCALCULATE -> (junction 14) [order 1] : [deltaV==0]
  SAMPLEandCALCULATE -> (junction 13) [order 2] : [deltaV~=0]
  (junction 13) -> DECREMENT_D [order 1] : [deltaI/deltaV>-Iavg/Vavg]
  (junction 13) -> RETURN [order 3] : [deltaI/deltaV==-Iavg/Vavg]
  (junction 13) -> INCREMENT_D [order 2] : [deltaI/deltaV<-Iavg/Vavg]
  (junction 14) -> INCREMENT_D [order 1] : [deltaI<0]
  (junction 14) -> RETURN [order 3] : [deltaI==0]
  (junction 14) -> DECREMENT_D [order 2] : [deltaI>0]
  DECREMENT_D -> RETURN
  INCREMENT_D -> RETURN
  data: deltaI local double; k local; deltaV local; Vavg input; Iavg input; Vprev input; Iprev input; d local double; D output
